simulink model "dsp_blr_8"  (R2018a)
settings: Solver=VariableStepAuto  StartTime=0.0  StopTime=100e-6  RelTol=1e-3
libraries: xbsIndex_r4 x60, xrbsSSR_Library x15, dspsigattribs x1, hdlsllib x1, simulink x1
(part 1 of 2)
settings Model: Creator=MoGURA  LastModifiedBy=1905p

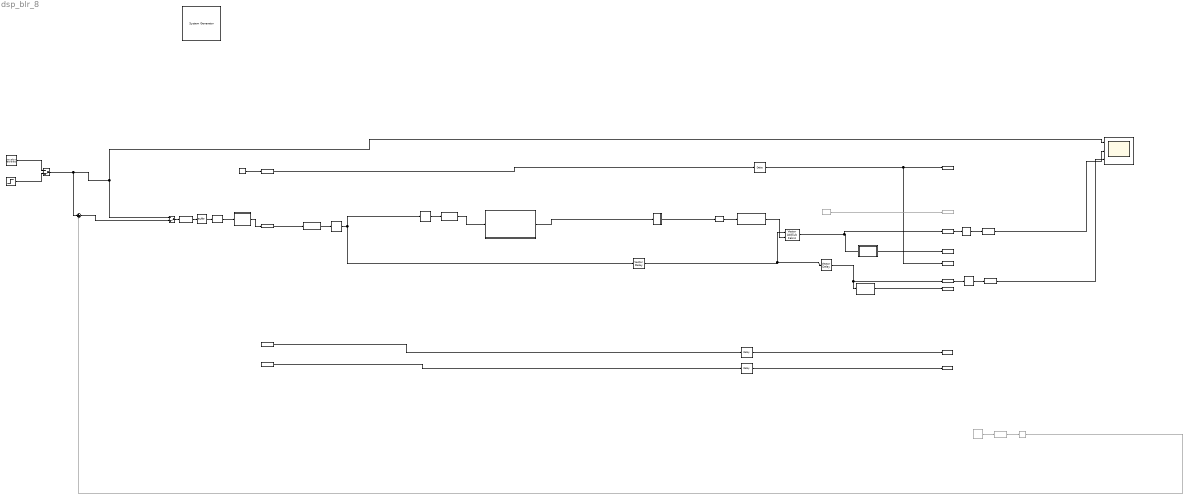
== system dsp_blr_8 ==
  note: 128bit
  note: DSP_module
  note: 16×8=128bit
      | のスカラー
  note: [a:b]を8個用意したが、[0:15]1個ではダメ?
      | 中身は全部同じだった
  note: 16bit
      | ...
      | 16bit
      | ↑
      | 8行のベクトル
  note: [a:b]とShiftで入力のvectorと同じ大きさになるようにした
  note: これを入れいるとなぜか上手くいく
  " System Generator" : xbsIndex_r4/ System Generator  Tag=genX  xilinxfamily=zynquplusRFSOC  part=xczu29dr  speed=-1-e  package=ffvf1760  synthesis_tool=Vivado  clock_wrapper=Clock Enables  directory=C:/Users/1905p/git_repos/KRD/ip_repos/SysGen_outputs/dsp_blr_8  proj_type=Vivado  Synth_file=Vivado Synthesis Defaults  Impl_file=Vivado Implementation Defaults  testbench=on  simulink_period=8e-9  sysclk_period=8  dcm_input_clock_period=10  incr_netlist=off  trim_vbits=Everywhere in SubSystem  dbl_ovrd=According to Block Masks  core_generation=According to Block Masks  run_coregen=off  deprecated_control=off  eval_field=0  block_type=sysgen
  +cut : Subsystem
  "?" : xbsIndex_r4/Convert  gui_display_data_type=Fixed-point  arith_type="Signed  (2's comp)"  n_bits=16  bin_pt=4  float_type=Single  exp_bits=8  fraction_bits=24  quantization=Truncate  overflow=Saturate  en=off  latency=1  pipeline=off  dbl_ovrd=off  block_type=convert
  Ave8 : Subsystem
  Buffer : Buffer  N=8  OutputFrames=off
  Convert 2-D to 1-D : dspsigattribs/Convert 2-D to 1-D
      settings: SourceProductName=DSP System Toolbox  SourceProductBaseCode=DS
  DBL_Scalar2Vector1 : Subsystem
  DIGITAL_BASELINE : xbsIndex_r4/Gateway Out  Commented=on  inherit_from_input=on  hdl_port=on  rows=1  columns=1  UseAsDAC=off  DACChannel='1'  interface=None  automatic_assignment=on  address_offset=hex2dec('00')  intf_name=''  intf_description=''  timing_constraint=None  locs_specified=off  LOCs={}  io_standard={}  block_type=gatewayout
  DSP_M_AXIS_TDATA : xbsIndex_r4/Gateway Out  inherit_from_input=on  hdl_port=on  rows=1  columns=1  UseAsDAC=off  DACChannel='1'  interface=None  automatic_assignment=on  address_offset=hex2dec('00')  intf_name=''  intf_description=''  timing_constraint=None  locs_specified=off  LOCs={}  io_standard={}  block_type=gatewayout
  DSP_M_AXIS_TDATA_debug : xrbsSSR_Library/Vector Real Gateway Out  inherit_from_input=on  hdl_port=off  rows=1  columns=1  UseAsDAC=off  DACChannel='1'  interface=None  automatic_assignment=on  address_offset=hex2dec('00')  intf_name=''  intf_description=''  timing_constraint=None  locs_specified=off  LOCs={}  io_standard={}  block_type=realgatewayout_ssr  sg_ssr=8  sg_ssr_prev=8  sg_ssr_name=vect_real_gwayout
      settings: SourceProductName=Xilinx SSR Blockset  infoedit=The Vector Real Gateway out block converts Xilinx fixed-point or floating-point type vector inputs into vector ouputs of type Simulink integer, single, double, or fixed-point.<br><br>Hardware notes: In hardware these blocks become top level output ports or are discarded, depending on how they are configured.
  DSP_M_AXIS_TVALID : xbsIndex_r4/Gateway Out  inherit_from_input=on  hdl_port=on  rows=1  columns=1  UseAsDAC=off  DACChannel='1'  interface=None  automatic_assignment=on  address_offset=hex2dec('00')  intf_name=''  intf_description=''  timing_constraint=None  locs_specified=off  LOCs={}  io_standard={}  block_type=gatewayout
  DSP_Vector2Scalar : Subsystem
  DSP_delay : xrbsSSR_Library/Vector Delay  sg_latency=7  infoeditControl=Selection of Reset will increase slice count due to use of real FFs and instead of SRLs  en=off  vectorize_en=off  rst=off  reg_retiming=off  block_type=delay_ssr  dbl_ovrd=off  sg_ssr=8  sg_ssr_prev=8  sg_ssr_name=vect_delay
      settings: SourceProductName=Xilinx SSR Blockset
  Delay : xbsIndex_r4/Delay  rst=off  infoeditControl=Selection of Reset will increase slice count due to use of real FFs and instead of SRLs  en=off  latency=7  reg_retiming=off  dbl_ovrd=off  block_type=delay
  HGAIN_Vector2Scalar : Subsystem
  HGAIN_delay : xrbsSSR_Library/Vector Delay  sg_latency=1  infoeditControl=Selection of Reset will increase slice count due to use of real FFs and instead of SRLs  en=off  vectorize_en=off  rst=off  reg_retiming=off  block_type=delay_ssr  dbl_ovrd=off  sg_ssr=8  sg_ssr_prev=8  sg_ssr_name=vect_delay
      settings: SourceProductName=Xilinx SSR Blockset
  H_M_AXIS_TDATA : xbsIndex_r4/Gateway Out  inherit_from_input=on  hdl_port=on  rows=1  columns=1  UseAsDAC=off  DACChannel='1'  interface=None  automatic_assignment=on  address_offset=hex2dec('00')  intf_name=''  intf_description=''  timing_constraint=None  locs_specified=off  LOCs={}  io_standard={}  block_type=gatewayout
  H_M_AXIS_TDATA_debug : xrbsSSR_Library/Vector Real Gateway Out  inherit_from_input=on  hdl_port=off  rows=1  columns=1  UseAsDAC=off  DACChannel='1'  interface=None  automatic_assignment=on  address_offset=hex2dec('00')  intf_name=''  intf_description=''  timing_constraint=None  locs_specified=off  LOCs={}  io_standard={}  block_type=realgatewayout_ssr  sg_ssr=8  sg_ssr_prev=8  sg_ssr_name=vect_real_gwayout
      settings: SourceProductName=Xilinx SSR Blockset  infoedit=The Vector Real Gateway out block converts Xilinx fixed-point or floating-point type vector inputs into vector ouputs of type Simulink integer, single, double, or fixed-point.<br><br>Hardware notes: In hardware these blocks become top level output ports or are discarded, depending on how they are configured.
  H_M_AXIS_TVALID : xbsIndex_r4/Gateway Out  inherit_from_input=on  hdl_port=on  rows=1  columns=1  UseAsDAC=off  DACChannel='1'  interface=None  automatic_assignment=on  address_offset=hex2dec('00')  intf_name=''  intf_description=''  timing_constraint=None  locs_specified=off  LOCs={}  io_standard={}  block_type=gatewayout
  H_S_AXIS_TDATA : xbsIndex_r4/Gateway In  gui_display_data_type=Fixed-point  arith_type=Unsigned  n_bits=128  bin_pt=0  preci_type=Single  exp_width=8  frac_width=24  rows=1  columns=1  quantization=Truncate  overflow=Wrap  period=8e-9  UseAsADC=off  ADCChannel='1'  interface=None  automatic_assignment=on  address_offset=hex2dec('00')  intf_name=''  intf_description=''  default_value=0  timing_constraint=None  locs_specified=off  LOCs={}  io_standard={}  inherit_from_input=off  hdl_port=on  dbl_ovrd=off  block_type=gatewayin
  H_S_AXIS_TVALID : xbsIndex_r4/Gateway In  gui_display_data_type=Boolean  arith_type=Boolean  n_bits=16  bin_pt=14  preci_type=Single  exp_width=8  frac_width=24  rows=1  columns=1  quantization="Round  (unbiased: +/- Inf)"  overflow=Saturate  period=8e-9  UseAsADC=off  ADCChannel='1'  interface=None  automatic_assignment=on  address_offset=hex2dec('00')  intf_name=''  intf_description=''  default_value=0  timing_constraint=None  locs_specified=off  LOCs={}  io_standard={}  inherit_from_input=off  hdl_port=on  dbl_ovrd=off  block_type=gatewayin
  L_GAIN_TDATA_delay : xbsIndex_r4/Delay  rst=off  infoeditControl=Selection of Reset will increase slice count due to use of real FFs and instead of SRLs  en=off  latency=0  reg_retiming=off  dbl_ovrd=off  block_type=delay
  L_GAIN_TVALID_delay : xbsIndex_r4/Delay  rst=off  infoeditControl=Selection of Reset will increase slice count due to use of real FFs and instead of SRLs  en=off  latency=0  reg_retiming=off  dbl_ovrd=off  block_type=delay
  L_M_AXIS_TDATA : xbsIndex_r4/Gateway Out  inherit_from_input=on  hdl_port=on  rows=1  columns=1  UseAsDAC=off  DACChannel='1'  interface=None  automatic_assignment=on  address_offset=hex2dec('00')  intf_name=''  intf_description=''  timing_constraint=None  locs_specified=off  LOCs={}  io_standard={}  block_type=gatewayout
  L_M_AXIS_TVALID : xbsIndex_r4/Gateway Out  inherit_from_input=on  hdl_port=on  rows=1  columns=1  UseAsDAC=off  DACChannel='1'  interface=None  automatic_assignment=on  address_offset=hex2dec('00')  intf_name=''  intf_description=''  timing_constraint=None  locs_specified=off  LOCs={}  io_standard={}  block_type=gatewayout
  L_S_AXIS_TDATA : xbsIndex_r4/Gateway In  gui_display_data_type=Fixed-point  arith_type=Unsigned  n_bits=32  bin_pt=0  preci_type=Single  exp_width=8  frac_width=24  rows=1  columns=1  quantization=Truncate  overflow=Wrap  period=8e-9  UseAsADC=off  ADCChannel='1'  interface=None  automatic_assignment=on  address_offset=hex2dec('00')  intf_name=''  intf_description=''  default_value=0  timing_constraint=None  locs_specified=off  LOCs={}  io_standard={}  inherit_from_input=off  hdl_port=on  dbl_ovrd=off  block_type=gatewayin
  L_S_AXIS_TVALID : xbsIndex_r4/Gateway In  gui_display_data_type=Boolean  arith_type=Boolean  n_bits=16  bin_pt=14  preci_type=Single  exp_width=8  frac_width=24  rows=1  columns=1  quantization="Round  (unbiased: +/- Inf)"  overflow=Saturate  period=8e-9  UseAsADC=off  ADCChannel='1'  interface=None  automatic_assignment=on  address_offset=hex2dec('00')  intf_name=''  intf_description=''  default_value=0  timing_constraint=None  locs_specified=off  LOCs={}  io_standard={}  inherit_from_input=off  hdl_port=on  dbl_ovrd=off  block_type=gatewayin
  Output data Type Conversion : DataTypeConversion  Commented=on  OutDataTypeStr=double
  Output data Type Conversion DSP : DataTypeConversion  OutDataTypeStr=double
  Output data Type Conversion HGAIN : DataTypeConversion  OutDataTypeStr=double
  Scalar2Vector : xrbsSSR_Library/Scalar2Vector  Width=16  sg_ssr=8  sg_ssr_prev=8  sg_ssr_name=vect_Scalar2Vector  block_type=scalar2vector_ssr
      settings: SourceProductName=Xilinx SSR Blockset
  Scope_xil : Scope  NumInputPorts=3
  Src Switch : ManualSwitch  CurrentSetting=0
  Src data Type Conversion : DataTypeConversion  OutMin=-2048  OutMax=2047  OutDataTypeStr=fixdt(1,16,4)
  Step : Step  Time=50e-6  After=-1024  SampleTime=1e-9
  Sum : Sum  Inputs=|+-
  Unbuffer : Unbuffer  Commented=on
  Unbuffer DSP : Unbuffer
  Unbuffer HGAIN : Unbuffer
  Vector AddSub Fabric2 : xrbsSSR_Library/Vector AddSub Fabric  mode=Subtraction  use_carryin=off  use_carryout=off  en=off  sg_latency=1  precision=User Defined  arith_type="Signed  (2's comp)"  n_bits=16  bin_pt=0  quantization=Truncate  overflow=Wrap  use_behavioral_HDL=off  hw_selection=Fabric  pipelined=off  dbl_ovrd=off  block_type=addsub_ssr  sg_ssr=8  sg_ssr_prev=8  sg_ssr_name=vect_addsubfab
      settings: SourceProductName=Xilinx SSR Blockset
  Vector Reinterpret : xrbsSSR_Library/Vector Reinterpret  sg_ssr=8  sg_ssr_prev=8  force_arith_type=on  arith_type="Signed  (2's comp)"  force_bin_pt=on  bin_pt=4  block_type=reinterpret_ssr
      settings: SourceProductName=Xilinx SSR Blockset  infoedit="The Vector Reinterpret block Changes vector input signal type without altering the binary representation. You can change the signal between signed and unsigned, and relocate the binary point.<br><br>Hardware notes: In hardware this block costs nothing.<br><br>Example:  Suppose the input is 6 bits wide, signed, with 2 fractional bits, and the output is forced to unsigned with 0 fractional bits.  Then an input of -2.0 (1110.00 in binary 2's complement) becomes an output of 56 (111000 in binary)."
  Vector Reinterpret2 : xrbsSSR_Library/Vector Reinterpret  sg_ssr=8  sg_ssr_prev=8  force_arith_type=on  arith_type=Unsigned  force_bin_pt=on  bin_pt=0  block_type=reinterpret_ssr
      settings: SourceProductName=Xilinx SSR Blockset  infoedit="The Vector Reinterpret block Changes vector input signal type without altering the binary representation. You can change the signal between signed and unsigned, and relocate the binary point.<br><br>Hardware notes: In hardware this block costs nothing.<br><br>Example:  Suppose the input is 6 bits wide, signed, with 2 fractional bits, and the output is forced to unsigned with 0 fractional bits.  Then an input of -2.0 (1110.00 in binary 2's complement) becomes an output of 56 (111000 in binary)."
  Vector2Bus : Subsystem
  Vector2Scalar1 : xrbsSSR_Library/Vector2Scalar  sg_ssr=8  sg_ssr_prev=8  sg_ssr_name=vect_Vector2Scalar  block_type=vector2scalar_ssr
      settings: SourceProductName=Xilinx SSR Blockset
  Waveform Generator : simulink/Sources/Waveform Generator  OutMin=[]  OutMax=[]  OutDataTypeStr=double  SelectedSignal=1  Signals=sin('Amplitude',1024,'Frequency',1000e3,'Phase',0)+square('Amplitude',400,'Frequency',20e6,'Phase',0,'DutyCycle',20)#pulse('Amplitude',1024,'TriggerTime',50e-9,'Duration',50e-9)+step('StepTime',100e-9,'InitialValue',0,'FinalValue',-512)  BlockNames=MultiportSwitch_2ee4ca9575f04b1#MultiportSwitch_74e4ddee714d4bc  SampleTime=1e-9
      settings: SourceProductName=Simulink
  blr_switch : ManualSwitch  CurrentSetting=0
  cast_DBL_out : xbsIndex_r4/Convert  Commented=on  gui_display_data_type=Fixed-point  arith_type="Signed  (2's comp)"  n_bits=16  bin_pt=0  float_type=Single  exp_bits=8  fraction_bits=24  quantization=Truncate  overflow=Wrap  en=off  latency=1  pipeline=off  dbl_ovrd=off  block_type=convert
  ext_delay : Delay  Commented=on  DelayLength=3  InitialCondition=0
  tvalid : Constant  VectorParams1D=off  OutDataTypeStr=Inherit: Inherit via back propagation  SampleTime=1/125e6
  wires:
  Src Switch/1 -> blr_switch/1, Scope_xil/1, Sum/1  "src_sig"
  ext_delay/1 -> Sum/2  "dac_out"
  Step/1 -> Src Switch/2
  Unbuffer/1 -> Output data Type Conversion/1
  Output data Type Conversion/1 -> ext_delay/1
  Sum/1 -> blr_switch/2  "corrected_out"
  Waveform Generator/1 -> Src Switch/1
  Src data Type Conversion/1 -> Buffer/1
  tvalid/1 -> H_S_AXIS_TVALID/1
  Output data Type Conversion DSP/1 -> Scope_xil/2  "dsp_data"
  Unbuffer DSP/1 -> Output data Type Conversion DSP/1
  Unbuffer HGAIN/1 -> Output data Type Conversion HGAIN/1
  Output data Type Conversion HGAIN/1 -> Scope_xil/3  "bypassed_data"
  Delay/1 -> DSP_M_AXIS_TVALID/1, H_M_AXIS_TVALID/1
  L_GAIN_TVALID_delay/1 -> L_M_AXIS_TVALID/1
  H_S_AXIS_TDATA/1 -> Scalar2Vector/1
  L_S_AXIS_TVALID/1 -> L_GAIN_TVALID_delay/1
  Buffer/1 -> Convert 2-D to 1-D/1
  Vector AddSub Fabric2/1 -> DSP_M_AXIS_TDATA_debug/1, DSP_Vector2Scalar/1(In1)
  DSP_M_AXIS_TDATA_debug/1 -> Unbuffer DSP/1
  H_M_AXIS_TDATA_debug/1 -> Unbuffer HGAIN/1
  L_S_AXIS_TDATA/1 -> L_GAIN_TDATA_delay/1
  DSP_delay/1 -> HGAIN_delay/1, Vector AddSub Fabric2/1
  L_GAIN_TDATA_delay/1 -> L_M_AXIS_TDATA/1
  cast_DBL_out/1 -> DIGITAL_BASELINE/1
  HGAIN_Vector2Scalar/1(Out1) -> H_M_AXIS_TDATA/1
  DSP_Vector2Scalar/1(Out1) -> DSP_M_AXIS_TDATA/1
  Scalar2Vector/1 -> Vector Reinterpret/1
  Convert 2-D to 1-D/1 -> Vector2Bus/1(In1)
  Vector2Bus/1(Out1) -> H_S_AXIS_TDATA/1
  blr_switch/1 -> Src data Type Conversion/1
  H_S_AXIS_TVALID/1 -> Delay/1
  Vector Reinterpret2/1 -> Vector2Scalar1/1
  Vector2Scalar1/1 -> Ave8/1(tdata_in)
  Vector Reinterpret/1 -> Vector Reinterpret2/1, DSP_delay/1
  Ave8/1(sum_data_out) -> +cut/1(In1)
  "?"/1 -> DBL_Scalar2Vector1/1(In1)
  +cut/1(Out1) -> "?"/1
  HGAIN_delay/1 -> H_M_AXIS_TDATA_debug/1, HGAIN_Vector2Scalar/1(In1)
  DBL_Scalar2Vector1/1(Out1) -> Vector AddSub Fabric2/2

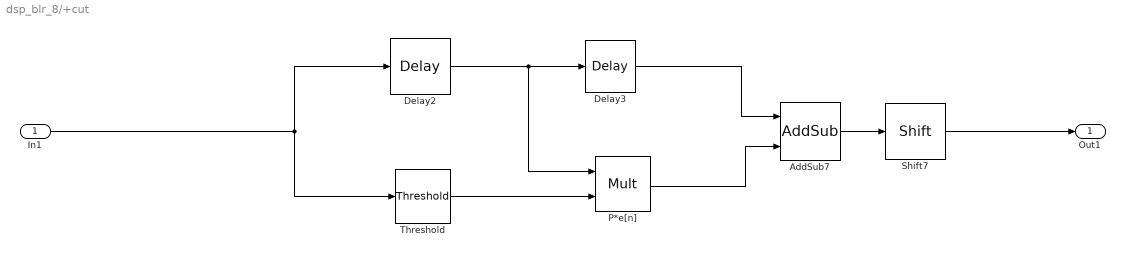
== system dsp_blr_8/+cut ==
  In1 : Inport
  AddSub7 : xbsIndex_r4/AddSub  mode=Subtraction  use_carryin=off  use_carryout=off  en=off  latency=0  precision=User Defined  arith_type="Signed  (2's comp)"  n_bits=17  bin_pt=4  quantization=Truncate  overflow=Wrap  use_behavioral_HDL=off  hw_selection=Fabric  pipelined=off  dbl_ovrd=off  block_type=addsub
  Delay2 : xbsIndex_r4/Delay  rst=off  infoeditControl=Selection of Reset will increase slice count due to use of real FFs and instead of SRLs  en=off  latency=1  reg_retiming=off  dbl_ovrd=off  block_type=delay
  Delay3 : xbsIndex_r4/Delay  rst=off  infoeditControl=Selection of Reset will increase slice count due to use of real FFs and instead of SRLs  en=off  latency=3  reg_retiming=off  dbl_ovrd=off  block_type=delay
  P*e[n] : xbsIndex_r4/Mult  precision=Full  arith_type="Signed  (2's comp)"  n_bits=16  bin_pt=14  quantization=Truncate  overflow=Wrap  en=off  latency=3  use_behavioral_HDL=off  opt=Speed  use_embedded=on  optimum_pipeline=off  pipeline=on  dbl_ovrd=off  use_rpm=on  placement_style=Triangular  block_type=mult
  Shift7 : xbsIndex_r4/Shift  shift_dir=Right  shift_bits=1  en=off  latency=1  precision=Full  arith_type="Signed  (2's comp)"  n_bits=16  bin_pt=14  quantization=Truncate  overflow=Wrap  dbl_ovrd=off  block_type=shift
  Threshold : xbsIndex_r4/Threshold  en=off  latency=1  dbl_ovrd=off  block_type=sgn
      settings: infoedit="Presents -1 as output if input is negative; otherwise presents 1.  Output is a two bit signed number."
  Out1 : Outport
  wires:
  Shift7/1 -> Out1/1
  Delay2/1 -> P*e[n]/1, Delay3/1
  In1/1 -> Threshold/1, Delay2/1
  Threshold/1 -> P*e[n]/2
  Delay3/1 -> AddSub7/1
  AddSub7/1 -> Shift7/1
  P*e[n]/1 -> AddSub7/2
